simulink model "mapp_4_fir_4_str"  (R2018b)
settings: Solver=ode45  StartTime=0.0  StopTime=200  RelTol=1e-3  EnableMultiTasking=on
undefined symbols (not defined in the file or in its folder): CMD_ci_Re_0, CMD_ci_Re_21, CMD_ci_str_0, CMD_ci_str_1, CMD_ci_str_10, CMD_ci_str_11, CMD_ci_str_12, CMD_ci_str_13, CMD_ci_str_14, CMD_ci_str_15, CMD_ci_str_16, CMD_ci_str_17, CMD_ci_str_18, CMD_ci_str_19, CMD_ci_str_2, CMD_ci_str_20, CMD_ci_str_21, CMD_ci_str_3, CMD_ci_str_4, CMD_ci_str_5, CMD_ci_str_6, CMD_ci_str_7, CMD_ci_str_8, CMD_ci_str_9, CMD_decr_0, CMD_deka_down, CMD_deka_up, CMD_fb, CMD_FB_mult, CMD_Firprg_0, CMD_Firprg_1, CMD_gain, CMD_ind_mult, CMD_ind_mult_1, CMD_ind_mult_2, CMD_ind_mult_3, CMD_ind_mult_4, CMD_ind_stuk, CMD_ind_vol, CMD_ind_vol_1, CMD_ind_vol_2, CMD_ind_vol_3, CMD_ind_vol_4, CMD_init_dac, CMD_init_sw, CMD_molot_string, CMD_nl, CMD_nl_sl, CMD_omega_0, CMD_out_vol, CMD_param_0, CMD_param_5, CMD_pedal, CMD_reset, CMD_rst, CMD_shape_0, CMD_step_down, CMD_step_up, CMD_str_svertk, ind_mult_0 ... (+10)
libraries: xbsIndex_r4 x3300
(part 10 of 16)

== system mapp_4_fir_4_str/mashinka_0/Force_str0/Delay_disp ==
  In1 : Inport
  Convert20 : xbsIndex_r4/Convert  gui_display_data_type=Fixed-point  arith_type="Signed  (2's comp)"  n_bits=24  bin_pt=23  float_type=Single  exp_bits=8  fraction_bits=24  quantization=Truncate  overflow=Wrap  en=off  latency=0  pipeline=off  dbl_ovrd=off  block_type=convert
  Convert4 : xbsIndex_r4/Convert  gui_display_data_type=Floating-point  arith_type=Floating-point  n_bits=16  bin_pt=14  float_type=Single  exp_bits=8  fraction_bits=24  quantization=Truncate  overflow=Wrap  en=off  latency=3  pipeline=off  dbl_ovrd=off  block_type=convert
  curr128 : xbsIndex_r4/Delay  rst=off  infoeditControl=Selection of Reset will increase slice count due to use of real FFs and instead of SRLs  en=off  latency=1  reg_retiming=on  dbl_ovrd=off  block_type=delay
      settings: xl_area=[16 32 0 0 0 0 0]  block_version=VER_STRING_GOES_HERE
  curr31 : xbsIndex_r4/Delay  rst=off  infoeditControl=Selection of Reset will increase slice count due to use of real FFs and instead of SRLs  en=off  latency=11  reg_retiming=on  dbl_ovrd=off  block_type=delay
      settings: xl_area=[16 32 0 0 0 0 0]  block_version=VER_STRING_GOES_HERE
  curr81 : xbsIndex_r4/Delay  rst=off  infoeditControl=Selection of Reset will increase slice count due to use of real FFs and instead of SRLs  en=off  latency=45  reg_retiming=on  dbl_ovrd=off  block_type=delay
      settings: xl_area=[17 33 0 33 0 0 0]  block_version=VER_STRING_GOES_HERE
  curr82 : xbsIndex_r4/Delay  rst=off  infoeditControl=Selection of Reset will increase slice count due to use of real FFs and instead of SRLs  en=off  latency=1  reg_retiming=on  dbl_ovrd=off  block_type=delay
      settings: xl_area=[16 32 0 0 0 0 0]  block_version=VER_STRING_GOES_HERE
  Out1 : Outport
  wires:
  curr128/1 -> Convert4/1
  In1/1 -> Convert20/1
  Convert4/1 -> curr82/1
  curr82/1 -> curr81/1
  curr31/1 -> Out1/1
  curr81/1 -> curr31/1
  Convert20/1 -> curr128/1

== system mapp_4_fir_4_str/mashinka_0/Force_str0/Delay_disp_decr ==
  In1 : Inport
  Convert3 : xbsIndex_r4/Convert  gui_display_data_type=Floating-point  arith_type=Floating-point  n_bits=16  bin_pt=14  float_type=Single  exp_bits=8  fraction_bits=24  quantization=Truncate  overflow=Wrap  en=off  latency=6  pipeline=off  dbl_ovrd=off  block_type=convert
  Convert39 : xbsIndex_r4/Convert  gui_display_data_type=Fixed-point  arith_type="Signed  (2's comp)"  n_bits=24  bin_pt=23  float_type=Single  exp_bits=8  fraction_bits=24  quantization=Truncate  overflow=Wrap  en=off  latency=0  pipeline=off  dbl_ovrd=off  block_type=convert
  Register73 : xbsIndex_r4/Register  init=0  rst=off  en=off  dbl_ovrd=off  block_type=register
  curr34 : xbsIndex_r4/Delay  rst=off  infoeditControl=Selection of Reset will increase slice count due to use of real FFs and instead of SRLs  en=off  latency=69  reg_retiming=on  dbl_ovrd=off  block_type=delay
      settings: xl_area=[17 33 0 33 0 0 0]  block_version=VER_STRING_GOES_HERE
  curr84 : xbsIndex_r4/Delay  rst=off  infoeditControl=Selection of Reset will increase slice count due to use of real FFs and instead of SRLs  en=off  latency=2  reg_retiming=on  dbl_ovrd=off  block_type=delay
      settings: xl_area=[17 33 0 33 0 0 0]  block_version=VER_STRING_GOES_HERE
  Out1 : Outport
  wires:
  Convert39/1 -> Register73/1
  curr34/1 -> curr84/1
  Register73/1 -> curr34/1
  In1/1 -> Convert39/1
  Convert3/1 -> Out1/1
  curr84/1 -> Convert3/1

== system mapp_4_fir_4_str/mashinka_0/Force_str0/Delay_level ==
  In1 : Inport
  Convert18 : xbsIndex_r4/Convert  gui_display_data_type=Fixed-point  arith_type="Signed  (2's comp)"  n_bits=32  bin_pt=24  float_type=Single  exp_bits=8  fraction_bits=24  quantization=Truncate  overflow=Wrap  en=off  latency=0  pipeline=off  dbl_ovrd=off  block_type=convert
  Convert19 : xbsIndex_r4/Convert  gui_display_data_type=Floating-point  arith_type=Floating-point  n_bits=ceil(log2(num_point_256-1));  bin_pt=0  float_type=Single  exp_bits=8  fraction_bits=24  quantization=Truncate  overflow=Wrap  en=off  latency=6  pipeline=off  dbl_ovrd=off  block_type=convert
  Delay{5,19,39..40} (4 alike) : xbsIndex_r4/Delay  rst=off  infoeditControl=Selection of Reset will increase slice count due to use of real FFs and instead of SRLs  en=off  latency=1  reg_retiming=off  dbl_ovrd=off  block_type=delay
  Delay38 : xbsIndex_r4/Delay  rst=off  infoeditControl=Selection of Reset will increase slice count due to use of real FFs and instead of SRLs  en=off  latency=88  reg_retiming=off  dbl_ovrd=off  block_type=delay
  Reinterpret1 : xbsIndex_r4/Reinterpret  force_arith_type=on  arith_type=Unsigned  force_bin_pt=on  bin_pt=21  block_type=cast
      settings: block_version=VER_STRING_GOES_HERE
  Out1 : Outport
  wires:
  Convert18/1 -> Delay19/1
  Reinterpret1/1 -> Delay5/1
  Delay38/1 -> Delay40/1
  Delay40/1 -> Reinterpret1/1
  In1/1 -> Delay39/1
  Delay5/1 -> Convert18/1
  Delay19/1 -> Convert19/1
  Convert19/1 -> Out1/1
  Delay39/1 -> Delay38/1

== system mapp_4_fir_4_str/mashinka_0/Force_str0/Delay_shape ==
  In1 : Inport
  Convert1 : xbsIndex_r4/Convert  gui_display_data_type=Floating-point  arith_type=Floating-point  n_bits=16  bin_pt=14  float_type=Single  exp_bits=8  fraction_bits=24  quantization=Truncate  overflow=Wrap  en=off  latency=6  pipeline=off  dbl_ovrd=off  block_type=convert
  Convert18 : xbsIndex_r4/Convert  gui_display_data_type=Fixed-point  arith_type="Signed  (2's comp)"  n_bits=24  bin_pt=23  float_type=Single  exp_bits=8  fraction_bits=24  quantization=Truncate  overflow=Wrap  en=off  latency=6  pipeline=off  dbl_ovrd=off  block_type=convert
  Register{1..2,49..50} (4 alike) : xbsIndex_r4/Register  init=0  rst=off  en=off  dbl_ovrd=off  block_type=register
  Reinterpret2 : xbsIndex_r4/Reinterpret  force_arith_type=on  arith_type="Signed  (2's comp)"  force_bin_pt=on  bin_pt=23  block_type=reinterpret
  curr16 : xbsIndex_r4/Delay  rst=off  infoeditControl=Selection of Reset will increase slice count due to use of real FFs and instead of SRLs  en=off  latency=9  reg_retiming=on  dbl_ovrd=off  block_type=delay
      settings: xl_area=[17 33 0 33 0 0 0]  block_version=VER_STRING_GOES_HERE
  Out1 : Outport
  wires:
  Register2/1 -> Out1/1
  Register1/1 -> Convert1/1
  In1/1 -> Reinterpret2/1
  curr16/1 -> Register50/1
  Reinterpret2/1 -> Register49/1
  Register50/1 -> Convert18/1
  Register49/1 -> curr16/1
  Convert18/1 -> Register1/1
  Convert1/1 -> Register2/1

== system mapp_4_fir_4_str/mashinka_0/Force_str0/Delay_thresh ==
  In1 : Inport
  Convert : xbsIndex_r4/Convert  gui_display_data_type=Fixed-point  arith_type="Signed  (2's comp)"  n_bits=32  bin_pt=24  float_type=Single  exp_bits=8  fraction_bits=24  quantization=Truncate  overflow=Wrap  en=off  latency=0  pipeline=off  dbl_ovrd=off  block_type=convert
  Convert14 : xbsIndex_r4/Convert  gui_display_data_type=Floating-point  arith_type=Floating-point  n_bits=ceil(log2(num_point_256-1));  bin_pt=0  float_type=Single  exp_bits=8  fraction_bits=24  quantization=Truncate  overflow=Wrap  en=off  latency=6  pipeline=off  dbl_ovrd=off  block_type=convert
  Delay{10,14,31..32} (4 alike) : xbsIndex_r4/Delay  rst=off  infoeditControl=Selection of Reset will increase slice count due to use of real FFs and instead of SRLs  en=off  latency=1  reg_retiming=off  dbl_ovrd=off  block_type=delay
  Delay29 : xbsIndex_r4/Delay  rst=off  infoeditControl=Selection of Reset will increase slice count due to use of real FFs and instead of SRLs  en=off  latency=45 - 2  reg_retiming=off  dbl_ovrd=off  block_type=delay
  Reinterpret5 : xbsIndex_r4/Reinterpret  force_arith_type=on  arith_type=Unsigned  force_bin_pt=on  bin_pt=21  block_type=cast
      settings: block_version=VER_STRING_GOES_HERE
  ttn_end : Outport
  wires:
  Delay31/1 -> Delay29/1
  Delay14/1 -> Convert14/1
  Delay32/1 -> Reinterpret5/1
  Delay10/1 -> Convert/1
  In1/1 -> Delay31/1
  Convert/1 -> Delay14/1
  Delay29/1 -> Delay32/1
  Reinterpret5/1 -> Delay10/1
  Convert14/1 -> ttn_end/1

== system mapp_4_fir_4_str/mashinka_0/Force_str0/Force_shape ==
  addr : Inport
  m_data : Inport  Port=2
  m_addr : Inport  Port=3
  m_en : Inport  Port=4
  Mux1 : xbsIndex_r4/Mux  inputs=2  en=off  latency=0  precision=Full  arith_type=Unsigned  n_bits=16  bin_pt=14  quantization=Truncate  overflow=Wrap  dbl_ovrd=off  block_type=mux
  Relational14 : xbsIndex_r4/Relational  mode=a=b  op_type=Bool  en=off  latency=0  dbl_ovrd=off  block_type=relational
  Single Port RAM2 : xbsIndex_r4/Single Port RAM  depth=256*2  initVector=shape2  distributed_mem=Block RAM  write_mode=Read After Write  rst=off  init_reg=0  en=off  latency=1  optimize=Area  dbl_ovrd=off  block_type=spram
  addr1 : xbsIndex_r4/Slice  nbits=9  boolean_output=off  mode=Lower Bit Location + Width  bit1=0  base1=MSB of Input  bit0=0  base0=LSB of Input  dbl_ovrd=off  block_type=slice
      settings: block_version=8.2-EVAL
  shape0 : xbsIndex_r4/Constant  const=shape0  gui_display_data_type=Fixed-point  arith_type=Unsigned  n_bits=8  bin_pt=0  preci_type=Single  exp_width=8  frac_width=24  explicit_period=on  period=1  equ=P=C  opselect=C  inp2=PCIN>>17  opr=+  inp1=P  carry=CIN  dbl_ovrd=off  block_type=constant
      settings: block_version=VER_STRING_GOES_HERE
  Out : Outport
  wires:
  Mux1/1 -> Single Port RAM2/1
  shape0/1 -> Relational14/2
  Relational14/1 -> Single Port RAM2/3, Mux1/1
  addr/1 -> Mux1/2
  m_en/1 -> Relational14/1
  Single Port RAM2/1 -> Out/1
  m_addr/1 -> addr1/1
  m_data/1 -> Single Port RAM2/2
  addr1/1 -> Mux1/3

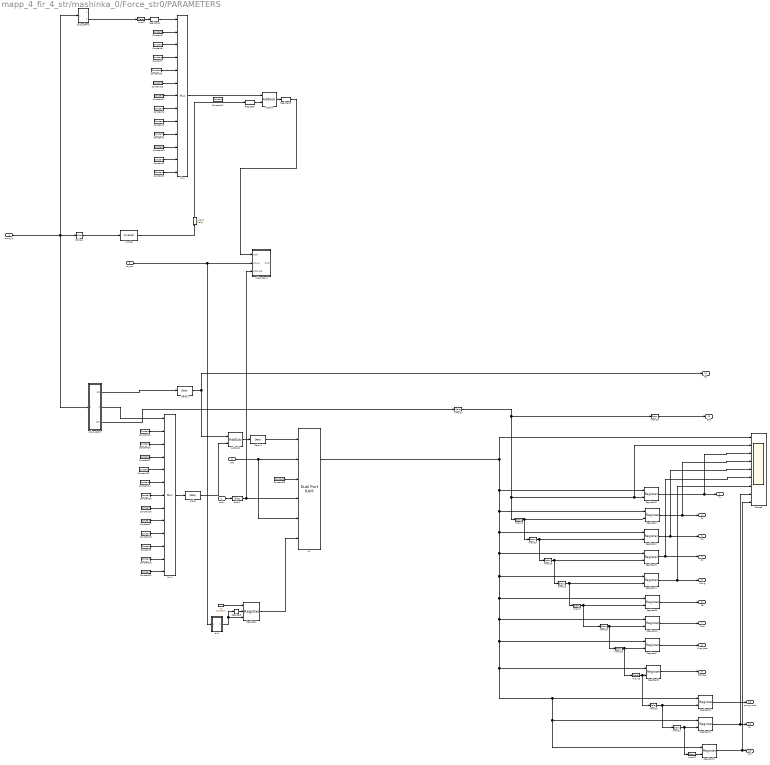
== system mapp_4_fir_4_str/mashinka_0/Force_str0/PARAMETERS ==
  addr : Inport
  dat : Inport  Port=2
  str_we : Inport  Port=3
  count_in : Inport  Port=4
  A1 : xbsIndex_r4/Dual Port RAM  depth=64  initVector=[(1:num_str1).*500 (1:num_str1).*8 (1:num_str1).*7 (1:num_str1).*6 200 300 400 500 (1:num_str1).*4 (1:num_str1).*70 (1:num_str1).*200 (1:num_str1).*10 (1:num_str1).*20 (1:num_str1).*0 (1:num_str1).*100]  distributed_mem=Block RAM  init_a=0  init_b=0  rst_a=off  rst_b=off  en_a=off  en_b=off  latency=2  write_mode_A=Read Before Write  write_mode_B=Read After Write  optimize=Speed  dbl_ovrd=off  block_type=dpram
      settings: xl_area=[0 0 3 0 0 0 0]  block_version=VER_STRING_GOES_HERE
  AddSub : xbsIndex_r4/AddSub  mode=Addition  use_carryin=off  use_carryout=off  en=off  latency=1  precision=User Defined  arith_type=Unsigned  n_bits=ceil(log2(num_param*num_str0))  bin_pt=0  quantization=Truncate  overflow=Wrap  use_behavioral_HDL=off  hw_selection=Fabric  pipelined=off  use_rpm=on  dbl_ovrd=off  block_type=addsub
      settings: block_version=10.1.3
  AddSub1 : xbsIndex_r4/AddSub  mode=Addition  use_carryin=off  use_carryout=off  en=off  latency=2  precision=User Defined  arith_type=Unsigned  n_bits=ceil(log2(num_param*num_str1))  bin_pt=0  quantization=Truncate  overflow=Wrap  use_behavioral_HDL=off  hw_selection=Fabric  pipelined=off  use_rpm=on  dbl_ovrd=off  block_type=addsub
      settings: block_version=10.1.3
  Constant1 : xbsIndex_r4/Constant  const=num_str1*6  gui_display_data_type=Fixed-point  arith_type=Unsigned  n_bits=ceil(log2(num_str1*6))+1  bin_pt=0  preci_type=Single  exp_width=8  frac_width=24  explicit_period=on  period=1  equ=P=C  opselect=C  inp2=PCIN>>17  opr=+  inp1=P  carry=CIN  dbl_ovrd=off  block_type=constant
      settings: block_version=VER_STRING_GOES_HERE
  Constant10 : xbsIndex_r4/Constant  const=num_str1*6  gui_display_data_type=Fixed-point  arith_type=Unsigned  n_bits=ceil(log2(num_str1*6))+1  bin_pt=0  preci_type=Single  exp_width=8  frac_width=24  explicit_period=on  period=1  equ=P=C  opselect=C  inp2=PCIN>>17  opr=+  inp1=P  carry=CIN  dbl_ovrd=off  block_type=constant
      settings: block_version=VER_STRING_GOES_HERE
  Constant11 : xbsIndex_r4/Constant  const=0  gui_display_data_type=Boolean  arith_type=Boolean  n_bits=9  bin_pt=0  preci_type=Single  exp_width=8  frac_width=24  explicit_period=on  period=1  equ=P=C  opselect=C  inp2=PCIN>>17  opr=+  inp1=P  carry=CIN  dbl_ovrd=off  block_type=constant
      settings: block_version=VER_STRING_GOES_HERE
  Constant12 : xbsIndex_r4/Constant  const=num_str1*3  gui_display_data_type=Fixed-point  arith_type=Unsigned  n_bits=ceil(log2(num_str1*2)) +1  bin_pt=0  preci_type=Single  exp_width=8  frac_width=24  explicit_period=on  period=1  equ=P=C  opselect=C  inp2=PCIN>>17  opr=+  inp1=P  carry=CIN  dbl_ovrd=off  block_type=constant
      settings: block_version=VER_STRING_GOES_HERE
  Constant13 : xbsIndex_r4/Constant  const=num_str1*4  gui_display_data_type=Fixed-point  arith_type=Unsigned  n_bits=ceil(log2(num_str1*4)) +1  bin_pt=0  preci_type=Single  exp_width=8  frac_width=24  explicit_period=on  period=1  equ=P=C  opselect=C  inp2=PCIN>>17  opr=+  inp1=P  carry=CIN  dbl_ovrd=off  block_type=constant
      settings: block_version=VER_STRING_GOES_HERE
  Constant14 : xbsIndex_r4/Constant  const=num_str1*5  gui_display_data_type=Fixed-point  arith_type=Unsigned  n_bits=ceil(log2(num_str1*5))  bin_pt=0  preci_type=Single  exp_width=8  frac_width=24  explicit_period=on  period=1  equ=P=C  opselect=C  inp2=PCIN>>17  opr=+  inp1=P  carry=CIN  dbl_ovrd=off  block_type=constant
      settings: block_version=VER_STRING_GOES_HERE
  Constant15 : xbsIndex_r4/Constant  const=num_str1*9  gui_display_data_type=Fixed-point  arith_type=Unsigned  n_bits=ceil(log2(num_str1*9)) +1  bin_pt=0  preci_type=Single  exp_width=8  frac_width=24  explicit_period=on  period=1  equ=P=C  opselect=C  inp2=PCIN>>17  opr=+  inp1=P  carry=CIN  dbl_ovrd=off  block_type=constant
      settings: block_version=VER_STRING_GOES_HERE
  Constant16 : xbsIndex_r4/Constant  const=0  gui_display_data_type=Fixed-point  arith_type=Unsigned  n_bits=4  bin_pt=0  preci_type=Single  exp_width=8  frac_width=24  explicit_period=on  period=1  equ=P=C  opselect=C  inp2=PCIN>>17  opr=+  inp1=P  carry=CIN  dbl_ovrd=off  block_type=constant
      settings: block_version=VER_STRING_GOES_HERE
  Constant17 : xbsIndex_r4/Constant  const=num_str1*7  gui_display_data_type=Fixed-point  arith_type=Unsigned  n_bits=ceil(log2(num_str1*7))+1  bin_pt=0  preci_type=Single  exp_width=8  frac_width=24  explicit_period=on  period=1  equ=P=C  opselect=C  inp2=PCIN>>17  opr=+  inp1=P  carry=CIN  dbl_ovrd=off  block_type=constant
      settings: block_version=VER_STRING_GOES_HERE
  Constant18 : xbsIndex_r4/Constant  const=num_str1*8  gui_display_data_type=Fixed-point  arith_type=Unsigned  n_bits=ceil(log2(num_str1*8)) +1  bin_pt=0  preci_type=Single  exp_width=8  frac_width=24  explicit_period=on  period=1  equ=P=C  opselect=C  inp2=PCIN>>17  opr=+  inp1=P  carry=CIN  dbl_ovrd=off  block_type=constant
      settings: block_version=VER_STRING_GOES_HERE
  Constant19 : xbsIndex_r4/Constant  const=num_str1*10  gui_display_data_type=Fixed-point  arith_type=Unsigned  n_bits=ceil(log2(num_str1*10)) +1  bin_pt=0  preci_type=Single  exp_width=8  frac_width=24  explicit_period=on  period=1  equ=P=C  opselect=C  inp2=PCIN>>17  opr=+  inp1=P  carry=CIN  dbl_ovrd=off  block_type=constant
      settings: block_version=VER_STRING_GOES_HERE
  Constant2 : xbsIndex_r4/Constant  const=0  gui_display_data_type=Fixed-point  arith_type=Unsigned  n_bits=4  bin_pt=0  preci_type=Single  exp_width=8  frac_width=24  explicit_period=on  period=1  equ=P=C  opselect=C  inp2=PCIN>>17  opr=+  inp1=P  carry=CIN  dbl_ovrd=off  block_type=constant
      settings: block_version=VER_STRING_GOES_HERE
  Constant20 : xbsIndex_r4/Constant  const=num_str1  gui_display_data_type=Fixed-point  arith_type=Unsigned  n_bits=4  bin_pt=0  preci_type=Single  exp_width=8  frac_width=24  explicit_period=on  period=1  equ=P=C  opselect=C  inp2=PCIN>>17  opr=+  inp1=P  carry=CIN  dbl_ovrd=off  block_type=constant
      settings: block_version=VER_STRING_GOES_HERE
  Constant21 : xbsIndex_r4/Constant  const=num_str1*2  gui_display_data_type=Fixed-point  arith_type=Unsigned  n_bits=ceil(log2(num_str1*2)) +1  bin_pt=0  preci_type=Single  exp_width=8  frac_width=24  explicit_period=on  period=1  equ=P=C  opselect=C  inp2=PCIN>>17  opr=+  inp1=P  carry=CIN  dbl_ovrd=off  block_type=constant
      settings: block_version=VER_STRING_GOES_HERE
  Constant22 : xbsIndex_r4/Constant  const=num_str1*11  gui_display_data_type=Fixed-point  arith_type=Unsigned  n_bits=ceil(log2(num_str1*11)) +1  bin_pt=0  preci_type=Single  exp_width=8  frac_width=24  explicit_period=on  period=1  equ=P=C  opselect=C  inp2=PCIN>>17  opr=+  inp1=P  carry=CIN  dbl_ovrd=off  block_type=constant
      settings: block_version=VER_STRING_GOES_HERE
  Constant23 : xbsIndex_r4/Constant  const=num_str1*3  gui_display_data_type=Fixed-point  arith_type=Unsigned  n_bits=ceil(log2(num_str1*2)) +1  bin_pt=0  preci_type=Single  exp_width=8  frac_width=24  explicit_period=on  period=1  equ=P=C  opselect=C  inp2=PCIN>>17  opr=+  inp1=P  carry=CIN  dbl_ovrd=off  block_type=constant
      settings: block_version=VER_STRING_GOES_HERE
  Constant24 : xbsIndex_r4/Constant  const=num_str1*4  gui_display_data_type=Fixed-point  arith_type=Unsigned  n_bits=ceil(log2(num_str1*4)) +1  bin_pt=0  preci_type=Single  exp_width=8  frac_width=24  explicit_period=on  period=1  equ=P=C  opselect=C  inp2=PCIN>>17  opr=+  inp1=P  carry=CIN  dbl_ovrd=off  block_type=constant
      settings: block_version=VER_STRING_GOES_HERE
  Constant25 : xbsIndex_r4/Constant  const=num_str1*5  gui_display_data_type=Fixed-point  arith_type=Unsigned  n_bits=ceil(log2(num_str1*5))  bin_pt=0  preci_type=Single  exp_width=8  frac_width=24  explicit_period=on  period=1  equ=P=C  opselect=C  inp2=PCIN>>17  opr=+  inp1=P  carry=CIN  dbl_ovrd=off  block_type=constant
      settings: block_version=VER_STRING_GOES_HERE
  Constant26 : xbsIndex_r4/Constant  const=0  gui_display_data_type=Boolean  arith_type=Boolean  n_bits=9  bin_pt=0  preci_type=Single  exp_width=8  frac_width=24  explicit_period=on  period=1  equ=P=C  opselect=C  inp2=PCIN>>17  opr=+  inp1=P  carry=CIN  dbl_ovrd=off  block_type=constant
      settings: block_version=VER_STRING_GOES_HERE
  Constant3 : xbsIndex_r4/Constant  const=num_str1*7  gui_display_data_type=Fixed-point  arith_type=Unsigned  n_bits=ceil(log2(num_str1*7))+1  bin_pt=0  preci_type=Single  exp_width=8  frac_width=24  explicit_period=on  period=1  equ=P=C  opselect=C  inp2=PCIN>>17  opr=+  inp1=P  carry=CIN  dbl_ovrd=off  block_type=constant
      settings: block_version=VER_STRING_GOES_HERE
  Constant4 : xbsIndex_r4/Constant  const=num_str1*8  gui_display_data_type=Fixed-point  arith_type=Unsigned  n_bits=ceil(log2(num_str1*8)) +1  bin_pt=0  preci_type=Single  exp_width=8  frac_width=24  explicit_period=on  period=1  equ=P=C  opselect=C  inp2=PCIN>>17  opr=+  inp1=P  carry=CIN  dbl_ovrd=off  block_type=constant
      settings: block_version=VER_STRING_GOES_HERE
  Constant5 : xbsIndex_r4/Constant  const=num_str1*10  gui_display_data_type=Fixed-point  arith_type=Unsigned  n_bits=ceil(log2(num_str1*10)) +1  bin_pt=0  preci_type=Single  exp_width=8  frac_width=24  explicit_period=on  period=1  equ=P=C  opselect=C  inp2=PCIN>>17  opr=+  inp1=P  carry=CIN  dbl_ovrd=off  block_type=constant
      settings: block_version=VER_STRING_GOES_HERE
  Constant6 : xbsIndex_r4/Constant  const=num_str1  gui_display_data_type=Fixed-point  arith_type=Unsigned  n_bits=4  bin_pt=0  preci_type=Single  exp_width=8  frac_width=24  explicit_period=on  period=1  equ=P=C  opselect=C  inp2=PCIN>>17  opr=+  inp1=P  carry=CIN  dbl_ovrd=off  block_type=constant
      settings: block_version=VER_STRING_GOES_HERE
  Constant7 : xbsIndex_r4/Constant  const=num_str1*2  gui_display_data_type=Fixed-point  arith_type=Unsigned  n_bits=ceil(log2(num_str1*2)) +1  bin_pt=0  preci_type=Single  exp_width=8  frac_width=24  explicit_period=on  period=1  equ=P=C  opselect=C  inp2=PCIN>>17  opr=+  inp1=P  carry=CIN  dbl_ovrd=off  block_type=constant
      settings: block_version=VER_STRING_GOES_HERE
  Constant8 : xbsIndex_r4/Constant  const=num_str1*11  gui_display_data_type=Fixed-point  arith_type=Unsigned  n_bits=ceil(log2(num_str1*11)) +1  bin_pt=0  preci_type=Single  exp_width=8  frac_width=24  explicit_period=on  period=1  equ=P=C  opselect=C  inp2=PCIN>>17  opr=+  inp1=P  carry=CIN  dbl_ovrd=off  block_type=constant
      settings: block_version=VER_STRING_GOES_HERE
  Constant9 : xbsIndex_r4/Constant  const=num_str1*9  gui_display_data_type=Fixed-point  arith_type=Unsigned  n_bits=ceil(log2(num_str1*9)) +1  bin_pt=0  preci_type=Single  exp_width=8  frac_width=24  explicit_period=on  period=1  equ=P=C  opselect=C  inp2=PCIN>>17  opr=+  inp1=P  carry=CIN  dbl_ovrd=off  block_type=constant
      settings: block_version=VER_STRING_GOES_HERE
  Delay : xbsIndex_r4/Delay  rst=off  infoeditControl=Selection of Reset will increase slice count due to use of real FFs and instead of SRLs  en=off  latency=1  reg_retiming=off  dbl_ovrd=off  block_type=delay
  Delay1 : xbsIndex_r4/Delay  rst=off  infoeditControl=Selection of Reset will increase slice count due to use of real FFs and instead of SRLs  en=off  latency=1  reg_retiming=off  dbl_ovrd=off  block_type=delay
  Delay2 : xbsIndex_r4/Delay  rst=off  infoeditControl=Selection of Reset will increase slice count due to use of real FFs and instead of SRLs  en=off  latency=1  reg_retiming=off  dbl_ovrd=off  block_type=delay
  Imax{16..26,28} (12 alike) : xbsIndex_r4/Delay  rst=off  infoeditControl=Selection of Reset will increase slice count due to use of real FFs and instead of SRLs  en=off  latency=1  reg_retiming=off  dbl_ovrd=off  block_type=delay
      Imax16 settings: infoedit=Hardware notes: A delay line is a chain, each link of which is an SRL16 followed by a flip-flop. If register retiming is enabled, the delay line is a chain of flip-flops.  xl_area=[1 1 0 1 0 0 0]  block_version=VER_STRING_GOES_HERE
      Imax17 settings: infoedit=Hardware notes: A delay line is a chain, each link of which is an SRL16 followed by a flip-flop. If register retiming is enabled, the delay line is a chain of flip-flops.  xl_area=[1 1 0 1 0 0 0]  block_version=VER_STRING_GOES_HERE
      Imax18 settings: infoedit=Hardware notes: A delay line is a chain, each link of which is an SRL16 followed by a flip-flop. If register retiming is enabled, the delay line is a chain of flip-flops.  xl_area=[1 1 0 1 0 0 0]  block_version=VER_STRING_GOES_HERE
      Imax19 settings: infoedit=Hardware notes: A delay line is a chain, each link of which is an SRL16 followed by a flip-flop. If register retiming is enabled, the delay line is a chain of flip-flops.  xl_area=[1 1 0 1 0 0 0]  block_version=VER_STRING_GOES_HERE
      Imax20 settings: infoedit=Hardware notes: A delay line is a chain, each link of which is an SRL16 followed by a flip-flop. If register retiming is enabled, the delay line is a chain of flip-flops.  xl_area=[1 1 0 1 0 0 0]  block_version=VER_STRING_GOES_HERE
      Imax21 settings: infoedit=Hardware notes: A delay line is a chain, each link of which is an SRL16 followed by a flip-flop. If register retiming is enabled, the delay line is a chain of flip-flops.  xl_area=[1 1 0 1 0 0 0]  block_version=VER_STRING_GOES_HERE
      Imax22 settings: infoedit=Hardware notes: A delay line is a chain, each link of which is an SRL16 followed by a flip-flop. If register retiming is enabled, the delay line is a chain of flip-flops.  xl_area=[1 1 0 1 0 0 0]  block_version=VER_STRING_GOES_HERE
      Imax23 settings: infoedit=Hardware notes: A delay line is a chain, each link of which is an SRL16 followed by a flip-flop. If register retiming is enabled, the delay line is a chain of flip-flops.  xl_area=[1 1 0 1 0 0 0]  block_version=VER_STRING_GOES_HERE
      Imax24 settings: infoedit=Hardware notes: A delay line is a chain, each link of which is an SRL16 followed by a flip-flop. If register retiming is enabled, the delay line is a chain of flip-flops.  xl_area=[1 1 0 1 0 0 0]  block_version=VER_STRING_GOES_HERE
      Imax25 settings: xl_area=[1 1 0 1 0 0 0]  block_version=VER_STRING_GOES_HERE
      Imax26 settings: infoedit=Hardware notes: A delay line is a chain, each link of which is an SRL16 followed by a flip-flop. If register retiming is enabled, the delay line is a chain of flip-flops.  xl_area=[1 1 0 1 0 0 0]  block_version=VER_STRING_GOES_HERE
      Imax28 settings: xl_area=[1 1 0 1 0 0 0]  block_version=VER_STRING_GOES_HERE
  Imax2 : xbsIndex_r4/Delay  rst=off  infoeditControl=Selection of Reset will increase slice count due to use of real FFs and instead of SRLs  en=off  latency=254  reg_retiming=off  dbl_ovrd=off  block_type=delay
      settings: xl_area=[1 1 0 1 0 0 0]  block_version=VER_STRING_GOES_HERE
  Imax27 : xbsIndex_r4/Delay  rst=off  infoeditControl=Selection of Reset will increase slice count due to use of real FFs and instead of SRLs  en=off  latency=6  reg_retiming=off  dbl_ovrd=off  block_type=delay
      settings: xl_area=[1 1 0 1 0 0 0]  block_version=VER_STRING_GOES_HERE
  Imax3 : xbsIndex_r4/Delay  rst=off  infoeditControl=Selection of Reset will increase slice count due to use of real FFs and instead of SRLs  en=off  latency=6  reg_retiming=off  dbl_ovrd=off  block_type=delay
      settings: xl_area=[1 1 0 1 0 0 0]  block_version=VER_STRING_GOES_HERE
  Inverter : xbsIndex_r4/Inverter  en=off  latency=0  dbl_ovrd=off  block_type=inv
  Mux : xbsIndex_r4/Mux  inputs=12  en=off  latency=0  precision=Full  arith_type=Unsigned  n_bits=16  bin_pt=14  quantization=Truncate  overflow=Wrap  dbl_ovrd=off  block_type=mux
  Mux1 : xbsIndex_r4/Mux  inputs=12  en=off  latency=0  precision=Full  arith_type=Unsigned  n_bits=16  bin_pt=14  quantization=Truncate  overflow=Wrap  dbl_ovrd=off  block_type=mux
  RSlice1 : xbsIndex_r4/Slice  nbits=ceil(log2(num_str1));  boolean_output=off  mode=Lower Bit Location + Width  bit1=0  base1=MSB of Input  bit0=ceil(log2(num_point_256))-1;  base0=LSB of Input  dbl_ovrd=off  block_type=slice
      settings: block_version=VER_STRING_GOES_HERE
  Register{5..6,10..11} (4 alike) : xbsIndex_r4/Register  init=0  rst=off  en=off  dbl_ovrd=off  block_type=register
  Register{16..27} (12 alike) : xbsIndex_r4/Register  init=0  rst=off  en=on  dbl_ovrd=off  block_type=register
  Register4 : xbsIndex_r4/Register  init=0  rst=on  en=on  dbl_ovrd=off  block_type=register
      settings: block_version=8.2-EVAL
  Scope3 : Scope  NumInputPorts=9
  Subsystem1 : Subsystem
  Subsystem2 : Subsystem
  Subsystem3 : Subsystem
  addr1 : xbsIndex_r4/Slice  nbits=ceil(log2(num_param*num_str1))  boolean_output=off  mode=Lower Bit Location + Width  bit1=0  base1=MSB of Input  bit0=0  base0=LSB of Input  dbl_ovrd=off  block_type=slice
      settings: block_version=8.2-EVAL
  en1 : Subsystem
  q : xbsIndex_r4/Constant  const=1  gui_display_data_type=Boolean  arith_type=Boolean  n_bits=8  bin_pt=0  preci_type=Single  exp_width=8  frac_width=24  explicit_period=on  period=1  equ=P=C  opselect=C  inp2=PCIN>>17  opr=+  inp1=P  carry=CIN  dbl_ovrd=off  block_type=constant
      settings: block_version=VER_STRING_GOES_HERE
  Tn : Outport
  Fo : Outport  Port=2
  Do : Outport  Port=3
  Dc : Outport  Port=4
  Sdvig : Outport  Port=5
  FB : Outport  Port=6
  Disp : Outport  Port=7
  Disp_decr : Outport  Port=8
  Damper : Outport  Port=9
  point_noise : Outport  Port=10
  NL : Outport  Port=11
  1-Nl : Outport  Port=12
  Strb : Outport  Port=13
  Acc : Outport  Port=14
  wires:
  Subsystem3/3(strb) -> Imax27/1
  Register5/1 -> Register4/2
  q/1 -> Register4/1
  en1/1(Out1) -> Register4/3, Register5/1
  RSlice1/1 -> Inverter/1
  Register11/1 -> Mux/1
  Imax3/1 -> Register11/1
  Register6/1 -> AddSub/2
  dat/1 -> A1/2, A1/5
  Subsystem2/2(Out1) -> Imax3/1
  addr/1 -> addr1/1
  str_we/1 -> Subsystem1/2(str_we), en1/1(In1)
  Mux/1 -> AddSub/1
  AddSub/1 -> Register10/1
  count_in/1 -> Subsystem2/1(In1), Subsystem3/1(count_in), RSlice1/1
  Register4/1 -> A1/6
  Imax2/1 -> Register6/1
  Inverter/1 -> Imax2/1
  Constant22/1 -> Mux1/13
  Constant19/1 -> Mux1/12
  Constant9/1 -> Mux1/11
  Constant18/1 -> Mux1/10
  Constant17/1 -> Mux1/9
  Constant10/1 -> Mux1/8
  Constant25/1 -> Mux1/7
  Constant24/1 -> Mux1/6
  Constant23/1 -> Mux1/5
  Constant21/1 -> Mux1/4
  Constant20/1 -> Mux1/3
  Constant16/1 -> Mux1/2
  Subsystem3/2(Out1) -> Mux1/1
  Mux1/1 -> Delay/1
  Subsystem3/1(acc) -> Delay1/1
  Delay/1 -> AddSub1/2
  Delay1/1 -> AddSub1/1, Acc/1
  Delay2/1 -> A1/1
  Constant26/1 -> A1/3
  AddSub1/1 -> Delay2/1
  addr1/1 -> Subsystem1/3(addr_prg), A1/4
  Register10/1 -> Subsystem1/1(addr)
  Imax20/1 -> Register20/2, Imax21/1
  Imax21/1 -> Register21/2, Imax22/1
  Imax22/1 -> Register19/2
  A1/1 -> Register17/1, Register22/1, Register23/1, Register26/1, Register27/1, Register18/1, Register19/1, Register21/1, Register20/1, Register25/1, Register24/1, Register16/1, Scope3/1
  Imax24/1 -> Imax25/1, Register17/2
  Imax19/1 -> Register18/2, Imax20/1
  Imax18/1 -> Imax19/1, Register27/2
  Imax23/1 -> Register26/2, Imax18/1
  Imax25/1 -> Imax26/1, Register22/2
  Imax26/1 -> Imax16/1, Register23/2
  Imax16/1 -> Imax17/1, Register24/2
  Imax17/1 -> Imax23/1, Register25/2
  Register16/1 -> Tn/1, Scope3/3
  Register17/1 -> Fo/1, Scope3/4
  Register22/1 -> Do/1, Scope3/5
  Register23/1 -> Dc/1, Scope3/6
  Imax27/1 -> Imax28/1, Scope3/2, Register16/2, Imax24/1
  Register19/1 -> 1-Nl/1, Scope3/9
  Register21/1 -> NL/1, Scope3/8
  Register20/1 -> point_noise/1
  Register18/1 -> Damper/1
  Register27/1 -> Disp_decr/1
  Register26/1 -> Disp/1
  Register25/1 -> FB/1
  Register24/1 -> Scope3/7, Sdvig/1
  Imax28/1 -> Strb/1
  Constant12/1 -> Mux/5
  Constant6/1 -> Mux/3
  Constant2/1 -> Mux/2
  Constant7/1 -> Mux/4
  Constant13/1 -> Mux/6
  Constant14/1 -> Mux/7
  Constant1/1 -> Mux/8
  Constant3/1 -> Mux/9
  Constant4/1 -> Mux/10
  Constant15/1 -> Mux/11
  Constant5/1 -> Mux/12
  Constant8/1 -> Mux/13
